simulink model "Engine"  (Simulink 9.2)
settings: Solver=ode23tb  StartTime=0.0  StopTime=50  FixedStep=0.001  EnableMultiTasking=on
values from neighbouring files (symbols this model uses):
  a0 = 1.1647e-05    [EngineData.m]
  a1 = 3.0718e-05    [EngineData.m]
  a2 = 0.0029    [EngineData.m]
  dP_thrREF = 10000    [EngineData.m]
  KpThr = 2.0000e-07    (= 2e-07)    [EngineData.m]
  KpWg = 2.0000e-07    (= 2e-07)    [EngineData.m]
  n_r = 2    [EngineData.m]
  r_c = 9.5000    (= 9.5)    [EngineData.m]
  T_z = [0 1 2 3 4 5 6 7 8 9 10 11 ... (401 elements, 401x1)]    [EUDC_MAN.mat]    (also in FTP75_MAN.mat = [0 1 2 3 4 5 6 7 8 9 10 11 ... (1875 elements, 1875x1)]; WLTP_MAN.mat = [0 1 2 3 4 5 6 7 8 9 10 11 ... (1801 elements, 1801x1)])
  TiThr = 1.0000e-04    (= 0.0001)    [EngineData.m]
  TiWg = 1.0000e-04    (= 0.0001)    [EngineData.m]
  toggle_paf = toggle(2)    [RunEngine.m]
  toggle_vol = toggle(3)    [RunEngine.m]
  toggle_Waf = toggle(4)    [RunEngine.m]
  toggle_Wc = toggle(5)    [RunEngine.m]
  toggle_Wic = toggle(6)    [RunEngine.m]
  toggle_Wth = toggle(7)    [RunEngine.m]
  toggle_xth = toggle(8)    [RunEngine.m]
  toggle_ypic = toggle(9)    [RunEngine.m]
  toggle_ypim = toggle(10)    [RunEngine.m]
  toggle_yTic = toggle(11)    [RunEngine.m]
  toggle_yWaf = toggle(12)    [RunEngine.m]
undefined symbols (not defined in the file or in its folder): Newton, Raphson, TC_ENGINE
libraries: simulink x3
(part 2 of 3)

== system Engine/Generic Single-Turbocharged Engine/Intake Manifold Control Volume ==
  note: Ideal Gas
      | Law
  note: Energy
      | Balance
  note: Mass
      | Balance
  note: p
  mFlow up : Inport
  T up : Inport  Port=2
  Q in : Inport  Port=3
  T down : Inport  Port=4
  mFlow down : Inport  Port=5
  Constant1 : Constant  Value=R
  Constant2 : Constant  Value=R
  Constant3 : Constant  Value=V
  H_in : Product  Inputs=3  SaturateOnIntegerOverflow=on  InputSameDT=on  OutDataTypeStr=Inherit: Same as first input
  H_out : Product  Inputs=3  SaturateOnIntegerOverflow=on  InputSameDT=on  OutDataTypeStr=Inherit: Same as first input
  H_out1 : Product  Inputs=*/  SaturateOnIntegerOverflow=on  InputSameDT=on  OutDataTypeStr=Inherit: Same as first input
  Receiver Mass : Integrator  InitialCondition=p_init*V/R/T_init  ZeroCross=off
  Receiver Temperature : Integrator  InitialCondition=T_init  ZeroCross=off
  Sum : Sum  Inputs=++|  SaturateOnIntegerOverflow=on  InputSameDT=on  OutDataTypeStr=Inherit: Same as first input
  Sum1 : Sum  Inputs=+-|  SaturateOnIntegerOverflow=on  InputSameDT=on  OutDataTypeStr=Inherit: Same as first input
  Sum2 : Sum  Inputs=+-+-  SaturateOnIntegerOverflow=on  InputSameDT=on  OutDataTypeStr=Inherit: Same as first input
  c_v : Constant  Value=R/(gamma-1)
  m*R*T/V : Product  Inputs=***/  SaturateOnIntegerOverflow=on  InputSameDT=on  OutDataTypeStr=Inherit: Same as first input
  m*c_v : Product  SaturateOnIntegerOverflow=on  InputSameDT=on  OutDataTypeStr=Inherit: Same as first input
  mFlow*c_v*T : Product  Inputs=3  SaturateOnIntegerOverflow=on  InputSameDT=on  OutDataTypeStr=Inherit: Same as first input
  T : Outport
  p : Outport  Port=2
  wires:
  mFlow*c_v*T/1 -> Sum2/4
  c_v/1 -> mFlow*c_v*T/1, m*c_v/1, Sum/2  "c_v"
  Sum1/1 -> mFlow*c_v*T/2, Receiver Mass/1
  Receiver Temperature/1 -> mFlow*c_v*T/3, m*R*T/V/1, T/1
  Constant2/1 -> m*R*T/V/2
  Constant3/1 -> m*R*T/V/4
  m*R*T/V/1 -> p/1
  H_out1/1 -> Receiver Temperature/1
  m*c_v/1 -> H_out1/2
  Sum2/1 -> H_out1/1
  Q in/1 -> Sum2/3
  H_out/1 -> Sum2/2
  H_in/1 -> Sum2/1
  mFlow up/1 -> Sum1/1, H_in/2
  mFlow down/1 -> H_out/2, Sum1/2
  T down/1 -> H_out/1
  T up/1 -> H_in/1
  Constant1/1 -> Sum/1
  Sum/1 -> H_out/3, H_in/3  "c_p"
  Receiver Mass/1 -> m*R*T/V/3, m*c_v/2

== system Engine/Generic Single-Turbocharged Engine/Intercooler Control Volume ==
  note: Ideal Gas
      | Law
  note: Energy
      | Balance
  note: Mass
      | Balance
  note: p
  mFlow up : Inport
  T up : Inport  Port=2
  Q in : Inport  Port=3
  T down : Inport  Port=4
  mFlow down : Inport  Port=5
  Constant1 : Constant  Value=R
  Constant2 : Constant  Value=R
  Constant3 : Constant  Value=V
  H_in : Product  Inputs=3  SaturateOnIntegerOverflow=on  InputSameDT=on  OutDataTypeStr=Inherit: Same as first input
  H_out : Product  Inputs=3  SaturateOnIntegerOverflow=on  InputSameDT=on  OutDataTypeStr=Inherit: Same as first input
  H_out1 : Product  Inputs=*/  SaturateOnIntegerOverflow=on  InputSameDT=on  OutDataTypeStr=Inherit: Same as first input
  Receiver Mass : Integrator  InitialCondition=p_init*V/R/T_init  ZeroCross=off
  Receiver Temperature : Integrator  InitialCondition=T_init  LowerSaturationLimit=0  ZeroCross=off
  Sum : Sum  Inputs=++|  SaturateOnIntegerOverflow=on  InputSameDT=on  OutDataTypeStr=Inherit: Same as first input
  Sum1 : Sum  Inputs=+-|  SaturateOnIntegerOverflow=on  InputSameDT=on  OutDataTypeStr=Inherit: Same as first input
  Sum2 : Sum  Inputs=+-+-  SaturateOnIntegerOverflow=on  InputSameDT=on  OutDataTypeStr=Inherit: Same as first input
  c_v : Constant  Value=R/(gamma-1)
  m*R*T/V : Product  Inputs=***/  SaturateOnIntegerOverflow=on  InputSameDT=on  OutDataTypeStr=Inherit: Same as first input
  m*c_v : Product  SaturateOnIntegerOverflow=on  InputSameDT=on  OutDataTypeStr=Inherit: Same as first input
  mFlow*c_v*T : Product  Inputs=3  SaturateOnIntegerOverflow=on  InputSameDT=on  OutDataTypeStr=Inherit: Same as first input
  T : Outport
  p : Outport  Port=2
  wires:
  mFlow*c_v*T/1 -> Sum2/4
  c_v/1 -> mFlow*c_v*T/1, m*c_v/1, Sum/2  "c_v"
  Sum1/1 -> mFlow*c_v*T/2, Receiver Mass/1
  Receiver Temperature/1 -> mFlow*c_v*T/3, m*R*T/V/1, T/1
  Constant2/1 -> m*R*T/V/2
  Constant3/1 -> m*R*T/V/4
  m*R*T/V/1 -> p/1
  H_out1/1 -> Receiver Temperature/1
  m*c_v/1 -> H_out1/2
  Sum2/1 -> H_out1/1
  Q in/1 -> Sum2/3
  H_out/1 -> Sum2/2
  H_in/1 -> Sum2/1
  mFlow up/1 -> Sum1/1, H_in/2
  mFlow down/1 -> H_out/2, Sum1/2
  T down/1 -> H_out/1
  T up/1 -> H_in/1
  Constant1/1 -> Sum/1
  Sum/1 -> H_out/3, H_in/3  "c_p"
  Receiver Mass/1 -> m*R*T/V/3, m*c_v/2

== system Engine/Generic Single-Turbocharged Engine/Intercooler Incompressible Restriction and Temperature model ==
  T_cool [K] : Inport
  p_up : Inport  Port=2
  T_up : Inport  Port=3
  T_down : Inport  Port=4
  p_down : Inport  Port=5
  Intercooler Temperature Simple : Subsystem  mask(Intercooler temperature){}
      mask help:
      | Intercooler temperature drop model using intercooler
      | efficiency, epsilon.
      |    T_out=T_in-epsilon*(T_in-T_cool)
      mask Help:
      | Enter the value for epsilon and the block will calculate
      | the temperature out for the
  Intercooler Flow : Subsystem  mask(Restriction Incompressible Flow){H=TC_ENGINE.interCooler.H, p_lin=TC_ENGINE.interCooler.p_lin}
      mask prompts: H "Flow resistance"; p_lin "Linearization limit [Pa]"
      mask help:
      | Flow restriction for incompressible flows.
      |
      | The flow is modelled using the following function for the pressure drop over the system where the conditions refer to upstream conditions.
      |
      | delta p=H mFlow^2 T_in/p_in
      mask Help:
      | <h3>Flow restriction for incompressible flows.</h3>
      | <br>
      | The flow is modelled using the following function for the pressure drop over the system where the conditions refer to upstream conditions.
      | <br>
      | delta p=H mFlow^2 T_in/p_in
  Saturation : Saturate  UpperLimit=1  LowerLimit=0  ZeroCross=off
  epsilon : Constant  Value=TC_ENGINE.interCooler.epsilon
  W_ic : Outport
  T_fwd_flow [K] : Outport  Port=2
  wires:
  Intercooler Flow/1(m flow) -> W_ic/1
  p_up/1 -> Intercooler Flow/1(p up)
  T_up/1 -> Intercooler Flow/2(T up)
  T_down/1 -> Intercooler Flow/3(T down)
  p_down/1 -> Intercooler Flow/4(p down)
  T_cool [K]/1 -> Intercooler Temperature Simple/2(T_cool)
  Intercooler Temperature Simple/1(T_out) -> T_fwd_flow [K]/1
  Intercooler Flow/2(T flow) -> Intercooler Temperature Simple/1(T_in)
  epsilon/1 -> Saturation/1  "epsilon"
  Saturation/1 -> Intercooler Temperature Simple/3(epsilon)

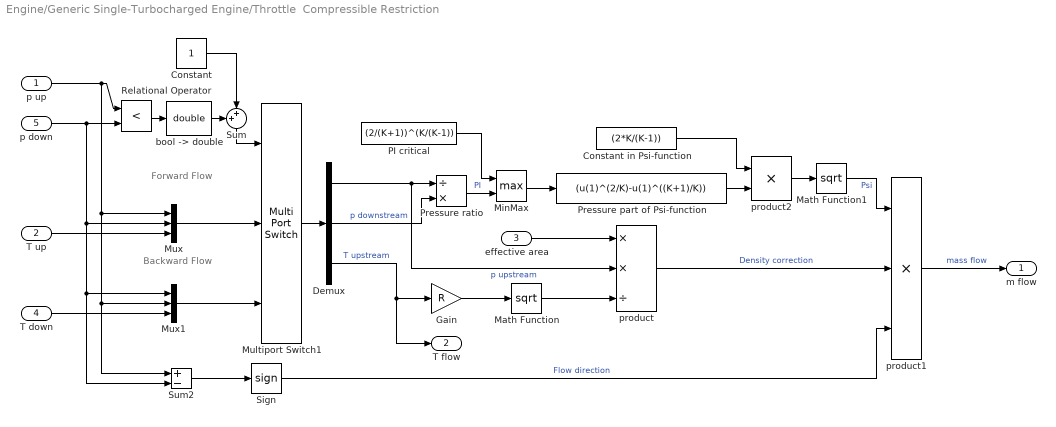
== system Engine/Generic Single-Turbocharged Engine/Throttle  Compressible Restriction ==
  note: Forward
      | Flow
  note: Backward
      | Flow
  p up : Inport
  T up : Inport  Port=2
  effective area : Inport  Port=3
  T down : Inport  Port=4
  p down : Inport  Port=5
  Constant : Constant
  Constant in Psi-function : Constant  Value=(2*K/(K-1))
  Demux : Demux  Outputs=3
  Gain : Gain  Gain=R  SaturateOnIntegerOverflow=on  OutDataTypeStr=Inherit: Same as input  ParamDataTypeStr=Inherit: Same as input
  Math Function : Math  Operator=sqrt  SaturateOnIntegerOverflow=on
  Math Function1 : Math  Operator=sqrt  SaturateOnIntegerOverflow=on
  MinMax : MinMax  Function=max  Inputs=2  ZeroCross=off  SaturateOnIntegerOverflow=on  InputSameDT=on
  Multiport Switch1 : MultiPortSwitch  Inputs=2  SaturateOnIntegerOverflow=on  InputSameDT=on
  Mux : Mux  Inputs=3
  Mux1 : Mux  Inputs=3
  PI critical : Constant  Value=(2/(K+1))^(K/(K-1))
  Pressure ratio : Product  Inputs=/*  SaturateOnIntegerOverflow=on  InputSameDT=on  OutDataTypeStr=Inherit: Same as first input
  Pressure part of Psi-function : Fcn  Expr=(u(1)^(2/K)-u(1)^((K+1)/K))
  Relational Operator : RelationalOperator  Operator=<  RndMeth=Nearest  InputSameDT=on
  Sign : Signum  ZeroCross=off
  Sum : Sum  Inputs=++|  SaturateOnIntegerOverflow=on  InputSameDT=on  OutDataTypeStr=Inherit: Same as first input
  Sum2 : Sum  Inputs=+-  SaturateOnIntegerOverflow=on  InputSameDT=on  OutDataTypeStr=Inherit: Same as first input
  "bool -> double" : DataTypeConversion  OutDataTypeStr=double  SaturateOnIntegerOverflow=on  RndMeth=Zero
  product : Product  Inputs=**/  SaturateOnIntegerOverflow=on  InputSameDT=on  OutDataTypeStr=Inherit: Same as first input
  product1 : Product  Inputs=3  SaturateOnIntegerOverflow=on  InputSameDT=on  OutDataTypeStr=Inherit: Same as first input
  product2 : Product  SaturateOnIntegerOverflow=on  InputSameDT=on  OutDataTypeStr=Inherit: Same as first input
  m flow : Outport
  T flow : Outport  Port=2
  wires:
  "bool -> double"/1 -> Sum/1
  Demux/3 -> T flow/1, Gain/1  "T upstream"
  Math Function1/1 -> product1/1  "Psi"
  product2/1 -> Math Function1/1
  Sign/1 -> product1/3  "Flow direction"
  product/1 -> product1/2  "Density correction"
  Pressure part of Psi-function/1 -> product2/2
  Constant in Psi-function/1 -> product2/1
  Math Function/1 -> product/3
  Gain/1 -> Math Function/1
  Demux/1 -> product/2, Pressure ratio/1  "p upstream"
  effective area/1 -> product/1
  product1/1 -> m flow/1  "mass flow"
  MinMax/1 -> Pressure part of Psi-function/1
  PI critical/1 -> MinMax/1
  Pressure ratio/1 -> MinMax/2  "PI"
  Sum2/1 -> Sign/1
  Demux/2 -> Pressure ratio/2  "p downstream"
  p up/1 -> Sum2/1, Mux1/2, Mux/1, Relational Operator/1
  p down/1 -> Sum2/2, Mux1/1, Mux/2, Relational Operator/2
  T up/1 -> Mux/3
  T down/1 -> Mux1/3
  Mux/1 -> Multiport Switch1/2
  Sum/1 -> Multiport Switch1/1
  Constant/1 -> Sum/2
  Mux1/1 -> Multiport Switch1/3
  Multiport Switch1/1 -> Demux/1
  Relational Operator/1 -> "bool -> double"/1

== system Engine/Generic Single-Turbocharged Engine/Turbine Control Volume ==
  note: Ideal Gas
      | Law
  note: Energy
      | Balance
  note: Mass
      | Balance
  note: p
  mFlow up : Inport
  T up : Inport  Port=2
  Q in : Inport  Port=3
  T down : Inport  Port=4
  mFlow down : Inport  Port=5
  Constant1 : Constant  Value=R
  Constant2 : Constant  Value=R
  Constant3 : Constant  Value=V
  H_in : Product  Inputs=3  SaturateOnIntegerOverflow=on  InputSameDT=on  OutDataTypeStr=Inherit: Same as first input
  H_out : Product  Inputs=3  SaturateOnIntegerOverflow=on  InputSameDT=on  OutDataTypeStr=Inherit: Same as first input
  H_out1 : Product  Inputs=*/  SaturateOnIntegerOverflow=on  InputSameDT=on  OutDataTypeStr=Inherit: Same as first input
  Receiver Mass : Integrator  InitialCondition=p_init*V/R/T_init  UpperSaturationLimit=500  LowerSaturationLimit=0  ZeroCross=off
  Receiver Temperature : Integrator  InitialCondition=T_init  UpperSaturationLimit=2000  LowerSaturationLimit=0  ZeroCross=off
  Sum : Sum  Inputs=++|  SaturateOnIntegerOverflow=on  InputSameDT=on  OutDataTypeStr=Inherit: Same as first input
  Sum1 : Sum  Inputs=+-|  SaturateOnIntegerOverflow=on  InputSameDT=on  OutDataTypeStr=Inherit: Same as first input
  Sum2 : Sum  Inputs=+-+-  SaturateOnIntegerOverflow=on  InputSameDT=on  OutDataTypeStr=Inherit: Same as first input
  c_v : Constant  Value=R/(gamma-1)
  m*R*T/V : Product  Inputs=***/  SaturateOnIntegerOverflow=on  InputSameDT=on  OutDataTypeStr=Inherit: Same as first input
  m*c_v : Product  SaturateOnIntegerOverflow=on  InputSameDT=on  OutDataTypeStr=Inherit: Same as first input
  mFlow*c_v*T : Product  Inputs=3  SaturateOnIntegerOverflow=on  InputSameDT=on  OutDataTypeStr=Inherit: Same as first input
  T : Outport
  p : Outport  Port=2
  wires:
  mFlow*c_v*T/1 -> Sum2/4
  c_v/1 -> mFlow*c_v*T/1, m*c_v/1, Sum/2  "c_v"
  Sum1/1 -> mFlow*c_v*T/2, Receiver Mass/1
  Receiver Temperature/1 -> mFlow*c_v*T/3, m*R*T/V/1, T/1
  Constant2/1 -> m*R*T/V/2
  Constant3/1 -> m*R*T/V/4
  m*R*T/V/1 -> p/1
  H_out1/1 -> Receiver Temperature/1
  m*c_v/1 -> H_out1/2
  Sum2/1 -> H_out1/1
  Q in/1 -> Sum2/3
  H_out/1 -> Sum2/2
  H_in/1 -> Sum2/1
  mFlow up/1 -> Sum1/1, H_in/2
  mFlow down/1 -> H_out/2, Sum1/2
  T down/1 -> H_out/1
  T up/1 -> H_in/1
  Constant1/1 -> Sum/1
  Sum/1 -> H_out/3, H_in/3  "c_p"
  Receiver Mass/1 -> m*R*T/V/3, m*c_v/2

== system Engine/Generic Single-Turbocharged Engine/Turbine and wastegate ==
  p_t : Inport
  T_t : Inport  Port=2
  w_tc : Inport  Port=3
  u_wg : Inport  Port=4
  p_em : Inport  Port=5
  T_em : Inport  Port=6
  A_wg : Gain  Gain=TC_ENGINE.wastegate.Amax*TC_ENGINE.wastegate.Cd  SaturateOnIntegerOverflow=on  OutDataTypeStr=Inherit: Same as input  ParamDataTypeStr=Inherit: Same as input
  A_wg2 : Gain  Gain=-1  SaturateOnIntegerOverflow=on  OutDataTypeStr=Inherit: Same as input  ParamDataTypeStr=Inherit: Same as input
  Adiabatic mixer : Subsystem  mask(Adiabatic mixer){c_p1=TC_ENGINE.gasProp.exh.cp, c_p2=TC_ENGINE.gasProp.exh.cp}
      mask prompts: c_p1 "Specific heats flow 1 [J/kg K]"; c_p2 "Specific heats flow 2 [J/kg K]"
  Turbine1 : Subsystem
  Wastegate : Subsystem  mask(Restriction - Compressible Flow){K=TC_ENGINE.gasProp.exh.kappa, R=TC_ENGINE.gasProp.exh.R}
      mask prompts: K "Ratio of specific heats"; R "Ideal gas constant [J/kg/ K]"
      mask help:
      | The flow is modelled using isentropic expansion in a nozzle with the assumption that there is no pressure recovery after the nozzle.
      |
      | See e.g. Heywood Appendix C for a derivation.
      mask Help:
      | <h3>Flow restriction for compressible flows.</h3>
      | <br>
      | The flow is modelled using isentropic expansion in a nozzle with the assumption that there is no pressure recovery after the nozzle.
      | 
      | See e.g. Heywood Appendix C for a derivation.
  T_turb : Outport
  W_es : Outport  Port=2
  Tq_t : Outport  Port=3
  wires:
  Wastegate/1(m flow) -> Adiabatic mixer/4(mFlow2)
  Wastegate/2(T flow) -> Adiabatic mixer/3(T2)
  A_wg/1 -> Wastegate/3(effective area)
  w_tc/1 -> Turbine1/1(w_tc [rad/s])
  p_t/1 -> Turbine1/2(p_t [Pa]), Wastegate/5(p down)
  p_em/1 -> Turbine1/3(p_em [Pa]), Wastegate/1(p up)
  T_em/1 -> Turbine1/4(T_em [K]), Wastegate/2(T up)
  u_wg/1 -> A_wg/1
  Adiabatic mixer/1(T mix) -> T_turb/1
  Adiabatic mixer/2(m tot) -> A_wg2/1
  Turbine1/3(W_t [kg/s]) -> Adiabatic mixer/2(mFlow1)
  Turbine1/1(Tq_t [Nm]) -> Tq_t/1
  Turbine1/2(T_t [K]) -> Adiabatic mixer/1(T1)
  T_t/1 -> Wastegate/4(T down)
  A_wg2/1 -> W_es/1

== system Engine/Generic Single-Turbocharged Engine/Waf Fault ==
  Tamb : Inport
  pamb : Inport  Port=2
  "pc " : Inport  Port=3
  Constant in Psi-function : Constant  Value=(2*K/(K-1))
  Manual Switch : ManualSwitch
  Math Function : Math  Operator=sqrt  SaturateOnIntegerOverflow=on
  Math Function1 : Math  SaturateOnIntegerOverflow=on
  MinMax : MinMax  Function=max  Inputs=2  ZeroCross=off  SaturateOnIntegerOverflow=on  InputSameDT=on
  PI critical : Constant  Value=(2/(K+1))^(K/(K-1))
  Pressure ratio : Product  Inputs=*/  SaturateOnIntegerOverflow=on  InputSameDT=on  OutDataTypeStr=Inherit: Same as first input
  Pressure part of Psi-function : Fcn  Expr=(u(1)^(2/K)-u(1)^((K+1)/K))
  Ramp : simulink/Sources/Ramp  slope=1/(2/3*T_z(end))  start=200  InitialOutput=0
  Saturation : Saturate  UpperLimit=inf  LowerLimit=0
  Step : Step  Time=0.3*size(T_z,1)  SampleTime=0
  To Workspace2 : ToWorkspace  VariableName=fWafSig  SaveFormat=Timeseries  SampleTime=-1
  product : Product  Inputs=*/*  SaturateOnIntegerOverflow=on  InputSameDT=on  OutDataTypeStr=Inherit: Same as first input
  product1 : Product  SaturateOnIntegerOverflow=on  InputSameDT=on  OutDataTypeStr=Inherit: Same as first input
  product2 : Product  SaturateOnIntegerOverflow=on  InputSameDT=on  OutDataTypeStr=Inherit: Same as first input
  "toggle " : Gain  Gain=toggle_Waf*10e-6  SaturateOnIntegerOverflow=on  OutDataTypeStr=Inherit: Same as input  ParamDataTypeStr=Inherit: Same as input
  fWaf : Outport
  wires:
  Tamb/1 -> Math Function/1  "T upstream"
  Math Function1/1 -> product1/1  "Psi"
  product2/1 -> Math Function1/1
  product/1 -> product1/2  "Density correction"
  Pressure part of Psi-function/1 -> product2/2
  Constant in Psi-function/1 -> product2/1
  pamb/1 -> Pressure ratio/1, product/1  "p upstream"
  MinMax/1 -> Pressure part of Psi-function/1
  PI critical/1 -> MinMax/1
  Pressure ratio/1 -> MinMax/2  "PI"
  Math Function/1 -> product/2
  "toggle "/1 -> product/3, To Workspace2/1
  "pc "/1 -> Pressure ratio/2
  product1/1 -> fWaf/1
  Ramp/1 -> Saturation/1
  Step/1 -> Manual Switch/2
  Saturation/1 -> Manual Switch/1
  Manual Switch/1 -> "toggle "/1

== system Engine/Generic Single-Turbocharged Engine/Wc Fault ==
  "pic " : Inport
  pamb : Inport  Port=2
  Tamb : Inport  Port=3
  Constant in Psi-function : Constant  Value=(2*K/(K-1))
  Math Function : Math  Operator=sqrt  SaturateOnIntegerOverflow=on
  Math Function1 : Math  Operator=sqrt  SaturateOnIntegerOverflow=on
  MinMax : MinMax  Function=max  Inputs=2  ZeroCross=off  SaturateOnIntegerOverflow=on  InputSameDT=on
  PI critical : Constant  Value=(2/(K+1))^(K/(K-1))
  Pressure ratio : Product  Inputs=*/  SaturateOnIntegerOverflow=on  InputSameDT=on  OutDataTypeStr=Inherit: Same as first input
  Pressure part of Psi-function : Fcn  Expr=(u(1)^(2/K)-u(1)^((K+1)/K))
  Step : Step  Time=0.4*size(T_z,1)  SampleTime=0
  To Workspace2 : ToWorkspace  VariableName=fWcSig  SaveFormat=Timeseries  SampleTime=-1
  product : Product  Inputs=*/*  SaturateOnIntegerOverflow=on  InputSameDT=on  OutDataTypeStr=Inherit: Same as first input
  product1 : Product  SaturateOnIntegerOverflow=on  InputSameDT=on  OutDataTypeStr=Inherit: Same as first input
  product2 : Product  SaturateOnIntegerOverflow=on  InputSameDT=on  OutDataTypeStr=Inherit: Same as first input
  "toggle " : Gain  Gain=toggle_Wc*3e-6  SaturateOnIntegerOverflow=on  OutDataTypeStr=Inherit: Same as input  ParamDataTypeStr=Inherit: Same as input
  fWc : Outport
  wires:
  Tamb/1 -> Math Function/1  "T upstream"
  Math Function1/1 -> product1/1  "Psi"
  product2/1 -> Math Function1/1
  product/1 -> product1/2  "Density correction"
  Pressure part of Psi-function/1 -> product2/2
  Constant in Psi-function/1 -> product2/1
  pamb/1 -> Pressure ratio/1, product/1  "p upstream"
  MinMax/1 -> Pressure part of Psi-function/1
  PI critical/1 -> MinMax/1
  Pressure ratio/1 -> MinMax/2  "PI"
  Math Function/1 -> product/2
  "toggle "/1 -> To Workspace2/1, product/3
  "pic "/1 -> Pressure ratio/2
  product1/1 -> fWc/1
  Step/1 -> "toggle "/1

== system Engine/Generic Single-Turbocharged Engine/Wic Fault ==
  "pic " : Inport
  pamb : Inport  Port=2
  Tamb : Inport  Port=3
  Constant in Psi-function : Constant  Value=(2*K/(K-1))
  Math Function : Math  Operator=sqrt  SaturateOnIntegerOverflow=on
  Math Function1 : Math  Operator=sqrt  SaturateOnIntegerOverflow=on
  MinMax : MinMax  Function=max  Inputs=2  ZeroCross=off  SaturateOnIntegerOverflow=on  InputSameDT=on
  PI critical : Constant  Value=(2/(K+1))^(K/(K-1))
  Pressure ratio : Product  Inputs=*/  SaturateOnIntegerOverflow=on  InputSameDT=on  OutDataTypeStr=Inherit: Same as first input
  Pressure part of Psi-function : Fcn  Expr=(u(1)^(2/K)-u(1)^((K+1)/K))
  Product1 : Product
  Step : Step  Time=0.4*size(T_z,1)  SampleTime=0
  Step1 : Step  Time=0.8*size(T_z,1)  Before=1  After=0  SampleTime=0
  To Workspace2 : ToWorkspace  VariableName=fWicSig  SaveFormat=Timeseries  SampleTime=-1
  product : Product  Inputs=*/*  SaturateOnIntegerOverflow=on  InputSameDT=on  OutDataTypeStr=Inherit: Same as first input
  product1 : Product  SaturateOnIntegerOverflow=on  InputSameDT=on  OutDataTypeStr=Inherit: Same as first input
  product2 : Product  SaturateOnIntegerOverflow=on  InputSameDT=on  OutDataTypeStr=Inherit: Same as first input
  "toggle " : Gain  Gain=toggle_Wic*10e-6  SaturateOnIntegerOverflow=on  OutDataTypeStr=Inherit: Same as input  ParamDataTypeStr=Inherit: Same as input
  fWic : Outport
  wires:
  Tamb/1 -> Math Function/1  "T upstream"
  Math Function1/1 -> product1/1  "Psi"
  product2/1 -> Math Function1/1
  product/1 -> product1/2  "Density correction"
  Pressure part of Psi-function/1 -> product2/2
  Constant in Psi-function/1 -> product2/1
  pamb/1 -> Pressure ratio/1, product/1  "p upstream"
  MinMax/1 -> Pressure part of Psi-function/1
  PI critical/1 -> MinMax/1
  Pressure ratio/1 -> MinMax/2  "PI"
  Math Function/1 -> product/2
  "toggle "/1 -> To Workspace2/1, product/3
  "pic "/1 -> Pressure ratio/2
  product1/1 -> fWic/1
  Product1/1 -> "toggle "/1
  Step/1 -> Product1/1
  Step1/1 -> Product1/2

== system Engine/Generic Single-Turbocharged Engine/Wth Fault ==
  pim : Inport
  Tamb : Inport  Port=2
  pamb : Inport  Port=3
  Constant in Psi-function : Constant  Value=(2*K/(K-1))
  Math Function : Math  Operator=sqrt  SaturateOnIntegerOverflow=on
  Math Function1 : Math  Operator=sqrt  SaturateOnIntegerOverflow=on
  MinMax : MinMax  Function=max  Inputs=2  ZeroCross=off  SaturateOnIntegerOverflow=on  InputSameDT=on
  PI critical : Constant  Value=(2/(K+1))^(K/(K-1))
  Pressure ratio : Product  Inputs=*/  SaturateOnIntegerOverflow=on  InputSameDT=on  OutDataTypeStr=Inherit: Same as first input
  Pressure part of Psi-function : Fcn  Expr=(u(1)^(2/K)-u(1)^((K+1)/K))
  Pulse Generator : DiscretePulseGenerator  PulseType=Time based  Period=200  PulseWidth=20  PhaseDelay=30
  To Workspace2 : ToWorkspace  VariableName=fWthSig  SaveFormat=Timeseries  SampleTime=-1
  product : Product  Inputs=*/*  SaturateOnIntegerOverflow=on  InputSameDT=on  OutDataTypeStr=Inherit: Same as first input
  product1 : Product  SaturateOnIntegerOverflow=on  InputSameDT=on  OutDataTypeStr=Inherit: Same as first input
  product2 : Product  SaturateOnIntegerOverflow=on  InputSameDT=on  OutDataTypeStr=Inherit: Same as first input
  "toggle " : Gain  Gain=toggle_Wth*1e-6  Multiplication=Matrix(K*u)  SaturateOnIntegerOverflow=on  OutDataTypeStr=Inherit: Same as input  ParamDataTypeStr=Inherit: Same as input
  fWth : Outport
  wires:
  Pulse Generator/1 -> "toggle "/1
  Tamb/1 -> Math Function/1  "T upstream"
  Math Function1/1 -> product1/1  "Psi"
  product2/1 -> Math Function1/1
  product/1 -> product1/2  "Density correction"
  Pressure part of Psi-function/1 -> product2/2
  Constant in Psi-function/1 -> product2/1
  pamb/1 -> Pressure ratio/2, product/1  "p upstream"
  MinMax/1 -> Pressure part of Psi-function/1
  PI critical/1 -> MinMax/1
  Pressure ratio/1 -> MinMax/2  "PI"
  Math Function/1 -> product/2
  "toggle "/1 -> To Workspace2/1, product/3
  pim/1 -> Pressure ratio/1
  product1/1 -> fWth/1

== system Engine/Generic Single-Turbocharged Engine/fyWaf Fault ==
  yWaf : Inport
  Product : Product
  Pulse Generator : DiscretePulseGenerator  PulseType=Time based  Period=150  PulseWidth=20  PhaseDelay=30
  Switch : Switch  Criteria=u2 > Threshold  ZeroCross=off
  To Workspace2 : ToWorkspace  VariableName=fyWafSig  SaveFormat=Timeseries  SampleTime=-1
  "toggle " : Gain  Gain=toggle_yWaf*1.2  SaturateOnIntegerOverflow=on  OutDataTypeStr=Inherit: Same as input  ParamDataTypeStr=Inherit: Same as input
  fyWaf : Outport
  wires:
  yWaf/1 -> Switch/3, Product/1
  "toggle "/1 -> Product/2, To Workspace2/1
  Pulse Generator/1 -> "toggle "/1
  Product/1 -> Switch/1, Switch/2
  Switch/1 -> fyWaf/1

== system Engine/Generic Single-Turbocharged Engine/yTic Fault ==
  yTic : Inport
  Pulse Generator : DiscretePulseGenerator  PulseType=Time based  Period=150  PulseWidth=20  PhaseDelay=30
  Sum : Sum  Inputs=|++
  To Workspace2 : ToWorkspace  VariableName=fyTicSig  SaveFormat=Timeseries  SampleTime=-1
  "toggle " : Gain  Gain=toggle_yTic*(-20)  SaturateOnIntegerOverflow=on  OutDataTypeStr=Inherit: Same as input  ParamDataTypeStr=Inherit: Same as input
  fyTic : Outport
  wires:
  yTic/1 -> Sum/1
  "toggle "/1 -> To Workspace2/1, Sum/2
  Pulse Generator/1 -> "toggle "/1
  Sum/1 -> fyTic/1

== system Engine/Generic Single-Turbocharged Engine/ypic Fault ==
  ypic : Inport
  Product : Product
  Pulse Generator : DiscretePulseGenerator  PulseType=Time based  Period=200  PulseWidth=20  PhaseDelay=30
  Switch : Switch  Criteria=u2 > Threshold  ZeroCross=off
  To Workspace2 : ToWorkspace  VariableName=fypicSig  SaveFormat=Timeseries  SampleTime=-1
  "toggle " : Gain  Gain=toggle_ypic*1.2  SaturateOnIntegerOverflow=on  OutDataTypeStr=Inherit: Same as input  ParamDataTypeStr=Inherit: Same as input
  fypic : Outport
  wires:
  ypic/1 -> Switch/3, Product/1
  "toggle "/1 -> Product/2, To Workspace2/1
  Product/1 -> Switch/1, Switch/2
  Switch/1 -> fypic/1
  Pulse Generator/1 -> "toggle "/1

== system Engine/Generic Single-Turbocharged Engine/ypim Fault ==
  ypim : Inport
  Manual Switch : ManualSwitch
  Product : Product
  Pulse Generator : DiscretePulseGenerator  PulseType=Time based  Period=120  PulseWidth=10  PhaseDelay=30
  Ramp : simulink/Sources/Ramp  slope=1/(2/3*T_z(end))  start=200  InitialOutput=0
  Saturation : Saturate  UpperLimit=inf  LowerLimit=0
  Switch : Switch  Criteria=u2 > Threshold  ZeroCross=off
  To Workspace2 : ToWorkspace  VariableName=fypimSig  SaveFormat=Timeseries  SampleTime=-1
  "toggle " : Gain  Gain=toggle_ypim*1.19  SaturateOnIntegerOverflow=on  OutDataTypeStr=Inherit: Same as input  ParamDataTypeStr=Inherit: Same as input
  fypim : Outport
  wires:
  ypim/1 -> Product/1, Switch/3
  "toggle "/1 -> Product/2, To Workspace2/1
  Product/1 -> Switch/1, Switch/2
  Switch/1 -> fypim/1
  Ramp/1 -> Saturation/1
  Pulse Generator/1 -> Manual Switch/2
  Saturation/1 -> Manual Switch/1
  Manual Switch/1 -> "toggle "/1

== system Engine/Boost Controller/Subsystem/% -> Area ==
  % : Inport
  Constant : Constant  Value=3
  Gain : Gain  Gain=997
  Sum : Sum  Inputs=|++
  A : Outport
  wires:
  Sum/1 -> A/1
  Constant/1 -> Sum/2
  Gain/1 -> Sum/1
  %/1 -> Gain/1

== system Engine/Boost Controller/Throttle Feed Forward /Aeff2alpha ==
  Aeff_REF : Inport
  AeffMinMax : Saturate  UpperLimit=a0+a1+a2  LowerLimit=a0
  Divide : Product  Inputs=*/
  Divide1 : Product  Inputs=/*/
  Sqrt : Sqrt  AlgorithmType=Newton-Raphson  SaturateOnIntegerOverflow=on
  Sub : Sum  Inputs=+-
  Sub1 : Sum
  Sub2 : Sum  Inputs=+-
  a0 : Constant  Value=a0
  a1 : Constant  Value=a1
  a2 : Constant  Value=a2
  square : Math  Operator=square  SaturateOnIntegerOverflow=on
  two : Constant  Value=2
  alpha_REF : Outport
  wires:
  Aeff_REF/1 -> AeffMinMax/1
  a0/1 -> Sub/2
  Sub/1 -> Divide/1
  a2/1 -> Divide/2, Divide1/1
  a1/1 -> Divide1/2
  two/1 -> Divide1/3
  Divide/1 -> Sub1/1
  Divide1/1 -> Sub2/2, square/1
  Sub1/1 -> Sqrt/1
  Sqrt/1 -> Sub2/1
  Sub2/1 -> alpha_REF/1
  square/1 -> Sub1/2
  AeffMinMax/1 -> Sub/1

== system Engine/Boost Controller/Throttle Feed Forward /Cylinder air flow REF ==
  p_im_REF : Inport
  T_im [K] : Inport  Port=2
  N [rad/s] : Inport  Port=3
  "p_em " : Inport  Port=4
  H_in2 : Product  Inputs=****/  SaturateOnIntegerOverflow=on  InputSameDT=on  OutDataTypeStr=Inherit: Same as first input
  Other constants : Constant  Value=V_D/4/pi/TC_ENGINE.gasProp.air.R
  Pressure ratio : Product  Inputs=/*  SaturateOnIntegerOverflow=on  InputSameDT=on  OutDataTypeStr=Inherit: Same as first input
  Sum : Sum  Inputs=+-|  SaturateOnIntegerOverflow=on  InputSameDT=on  OutDataTypeStr=Inherit: Same as first input
  Volumetric efficiency constants : Constant  Value=0.8/(r_c-1)
  compression ratio : Constant  Value=r_c
  expansion : Fcn  Expr=u(1)^(1/TC_ENGINE.gasProp.exh.kappa)
  product of constants : Product  SaturateOnIntegerOverflow=on  InputSameDT=on  OutDataTypeStr=Inherit: Same as first input
  m_dot_ac_REF : Outport
  wires:
  "p_em "/1 -> Pressure ratio/2
  expansion/1 -> Sum/2
  Pressure ratio/1 -> expansion/1  "PI"
  p_im_REF/1 -> H_in2/1, Pressure ratio/1
  Sum/1 -> H_in2/2
  product of constants/1 -> H_in2/3
  N [rad/s]/1 -> H_in2/4
  T_im [K]/1 -> H_in2/5
  Other constants/1 -> product of constants/2
  Volumetric efficiency constants/1 -> product of constants/1
  compression ratio/1 -> Sum/1
  H_in2/1 -> m_dot_ac_REF/1

== system Engine/Boost Controller/Throttle Feed Forward /Psi(PI) ==
  PI : Inport
  (g+1)/g : Constant  Value=(TC_ENGINE.throttle.gamma+1)/TC_ENGINE.throttle.gamma
  2/g : Constant  Value=2/TC_ENGINE.throttle.gamma
  2g/(g-1) : Constant  Value=(2*TC_ENGINE.throttle.gamma)/(TC_ENGINE.throttle.gamma-1)
  DivZeroProtect : MinMax  Function=max  Inputs=2
  Math Function : Math  Operator=pow  SaturateOnIntegerOverflow=on
  Math Function1 : Math  Operator=pow  SaturateOnIntegerOverflow=on
  MinMax : MinMax  Function=max  Inputs=2
  PI critical (2/(g+1))^(g/(g-1)) : Constant  Value=(2/(TC_ENGINE.throttle.gamma+1))^(TC_ENGINE.throttle.gamma/(TC_ENGINE.throttle.gamma-1))
  Product : Product  RndMeth=Zero
  Sqrt : Sqrt  AlgorithmType=Newton-Raphson  SaturateOnIntegerOverflow=on
  Subtract : Sum  Inputs=+-
  "[0,1]" : Saturate  UpperLimit=1  LowerLimit=0
  eps : Constant  Value=eps
  Psi : Outport
  wires:
  PI/1 -> "[0,1]"/1  "PI"
  PI critical (2/(g+1))^(g/(g-1))/1 -> MinMax/2
  MinMax/1 -> Math Function/1, Math Function1/1  "PIlim"
  2/g/1 -> Math Function/2
  (g+1)/g/1 -> Math Function1/2
  "[0,1]"/1 -> MinMax/1
  Math Function/1 -> Subtract/1
  Math Function1/1 -> Subtract/2
  Subtract/1 -> Product/1
  2g/(g-1)/1 -> Product/2
  Product/1 -> Sqrt/1
  Sqrt/1 -> DivZeroProtect/1  "Psi"
  eps/1 -> DivZeroProtect/2
  DivZeroProtect/1 -> Psi/1

== system Engine/Generic Single-Turbocharged Engine/Air filter Incompressible Restriction/paf Fault ==
  H : Inport
  H_in2 : Product  SaturateOnIntegerOverflow=on  InputSameDT=on  OutDataTypeStr=Inherit: Same as first input
  Manual Switch : ManualSwitch
  Ramp : simulink/Sources/Ramp  slope=1/(2/3*T_z(end))  start=200  InitialOutput=0
  Saturation : Saturate  UpperLimit=inf  LowerLimit=0
  Step : Step  Time=0.15*size(T_z,1)  SampleTime=0
  Switch : Switch  Criteria=u2 > Threshold  ZeroCross=off
  To Workspace2 : ToWorkspace  VariableName=fpafSig  SaveFormat=Timeseries  SampleTime=-1
  "toggle " : Gain  Gain=toggle_paf*80  SaturateOnIntegerOverflow=on  OutDataTypeStr=Inherit: Same as input  ParamDataTypeStr=Inherit: Same as input
  fpaf : Outport
  wires:
  H_in2/1 -> To Workspace2/1, Switch/2, Switch/1
  H/1 -> Switch/3, H_in2/1
  Switch/1 -> fpaf/1
  "toggle "/1 -> H_in2/2
  Ramp/1 -> Saturation/1
  Step/1 -> Manual Switch/2
  Saturation/1 -> Manual Switch/1
  Manual Switch/1 -> "toggle "/1

== system Engine/Generic Single-Turbocharged Engine/Compressor/Compressor Example ==
  note: Downstream temperature is included
      | to give the same interface as an
      | implementation of surge capable
      | compressor model.
  p_af [Pa] : Inport
  T_in [K] : Inport  Port=2
  w_tc [rad/s] : Inport  Port=3
  T_ds : Inport  Port=4
  p_c [Pa] : Inport  Port=5
  Compressor Efficiency : Subsystem
  Compressor Mass Flow : Subsystem
  Compressor Temperature : Subsystem  mask(Compressor Temperature){gamma_c=1.4}
      mask prompts: gamma_c "Compressor gamma [-]"
      mask help:
      | Compressor temperature increase.
      | It is determined directly from the definition compressor
      | efficiency.
      mask Help:
      | Enter the value for the ratio of specific heat
      | for the compressor.
  Compressor Torque : Subsystem  mask(Compressor Torque){c_p=1100}
      mask prompts: c_p "Compressor c_p [J/kg K]"
      mask help:
      | Calculates the compressor torque.
      | It is calculated using the control volume analysis of a
      | compressor, where it is assumed that c_p is constant for
      | the compression process.
      mask Help: Enter the value for the specific heat c_p in the dialog box.
  PI-calc : Subsystem
  Terminator : Terminator
  W_c : Outport
  T_c [K] : Outport  Port=2
  Tq_c [Nm] : Outport  Port=3
  wires:
  T_ds/1 -> Terminator/1
  Compressor Torque/1(Tq_c) -> Tq_c [Nm]/1
  Compressor Temperature/1(T_out) -> T_c [K]/1, Compressor Torque/4(T_out)
  PI-calc/1(PI) -> Compressor Temperature/3(Pi_c)  "PI_c"
  p_af [Pa]/1 -> Compressor Mass Flow/2(p_in [Pa]), PI-calc/1(p_af), Compressor Efficiency/3(p_in [Pa])
  p_c [Pa]/1 -> PI-calc/2(p_c), Compressor Mass Flow/4(p_c [Pa])
  T_in [K]/1 -> Compressor Efficiency/4(T_in [K]), Compressor Temperature/2(T_in), Compressor Torque/3(T_in), Compressor Mass Flow/3(T_in [K])
  w_tc [rad/s]/1 -> Compressor Mass Flow/1(w_c [rad/s]), Compressor Efficiency/1(w_c [rad/s]), Compressor Torque/1(omega_c)
  Compressor Mass Flow/1(W_c) -> W_c/1, Compressor Efficiency/2(W_c [kg/s]), Compressor Torque/2(mFlow_c)
  Compressor Efficiency/1(eta_c) -> Compressor Temperature/1(eta_c)

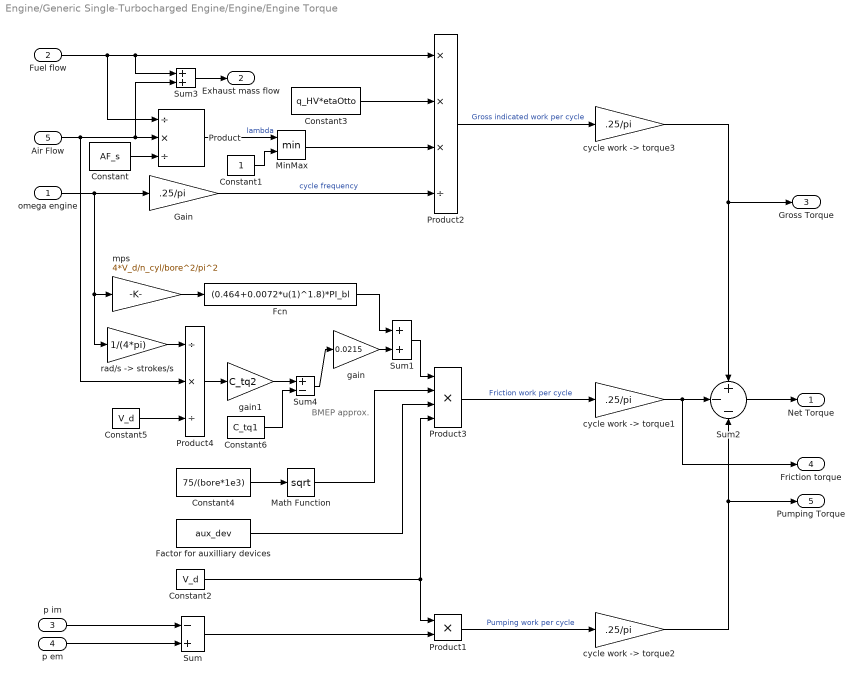
== system Engine/Generic Single-Turbocharged Engine/Engine/Engine Torque ==
  note: BMEP
      | approx.
  omega engine : Inport
  Fuel flow : Inport  Port=2
  p im : Inport  Port=3
  p em : Inport  Port=4
  Air Flow : Inport  Port=5
  Constant : Constant  Value=AF_s
  Constant1 : Constant
  Constant2 : Constant  Value=V_d
  Constant3 : Constant  Value=q_HV*etaOtto
  Constant4 : Constant  Value=75/(bore*1e3)
  Constant5 : Constant  Value=V_d
  Constant6 : Constant  Value=C_tq1
  Factor for auxilliary devices : Constant  Value=aux_dev
  Fcn : Fcn  Expr=(0.464+0.0072*u(1)^1.8)*PI_bl
  Gain : Gain  Gain=.25/pi  SaturateOnIntegerOverflow=on  OutDataTypeStr=Inherit: Same as input  ParamDataTypeStr=Inherit: Same as input
  Math Function : Math  Operator=sqrt  SaturateOnIntegerOverflow=on
  MinMax : MinMax  Inputs=2  ZeroCross=off  SaturateOnIntegerOverflow=on  InputSameDT=on
  Product : Product  Inputs=/*/  SaturateOnIntegerOverflow=on  InputSameDT=on  OutDataTypeStr=Inherit: Same as first input
  Product1 : Product  SaturateOnIntegerOverflow=on  InputSameDT=on  OutDataTypeStr=Inherit: Same as first input
  Product2 : Product  Inputs=***/  SaturateOnIntegerOverflow=on  InputSameDT=on  OutDataTypeStr=Inherit: Same as first input
  Product3 : Product  Inputs=4  SaturateOnIntegerOverflow=on  InputSameDT=on  OutDataTypeStr=Inherit: Same as first input
  Product4 : Product  Inputs=/*/  SaturateOnIntegerOverflow=on  InputSameDT=on  OutDataTypeStr=Inherit: Same as first input
  Sum : Sum  Inputs=-+  SaturateOnIntegerOverflow=on  InputSameDT=on  OutDataTypeStr=Inherit: Same as first input
  Sum1 : Sum  Inputs=2  SaturateOnIntegerOverflow=on  InputSameDT=on  OutDataTypeStr=Inherit: Same as first input
  Sum2 : Sum  Inputs=+--  SaturateOnIntegerOverflow=on  InputSameDT=on  OutDataTypeStr=Inherit: Same as first input
  Sum3 : Sum  Inputs=2  SaturateOnIntegerOverflow=on  InputSameDT=on  OutDataTypeStr=Inherit: Same as first input
  Sum4 : Sum  Inputs=+-  SaturateOnIntegerOverflow=on  InputSameDT=on  OutDataTypeStr=Inherit: Same as first input
  "cycle work -> torque1" : Gain  Gain=.25/pi  SaturateOnIntegerOverflow=on  OutDataTypeStr=Inherit: Same as input  ParamDataTypeStr=Inherit: Same as input
  "cycle work -> torque2" : Gain  Gain=.25/pi  SaturateOnIntegerOverflow=on  OutDataTypeStr=Inherit: Same as input  ParamDataTypeStr=Inherit: Same as input
  "cycle work -> torque3" : Gain  Gain=.25/pi  SaturateOnIntegerOverflow=on  OutDataTypeStr=Inherit: Same as input  ParamDataTypeStr=Inherit: Same as input
  gain : Gain  Gain=0.0215  SaturateOnIntegerOverflow=on  OutDataTypeStr=Inherit: Same as input  ParamDataTypeStr=Inherit: Same as input
  gain1 : Gain  Gain=C_tq2  SaturateOnIntegerOverflow=on  OutDataTypeStr=Inherit: Same as input  ParamDataTypeStr=Inherit: Same as input
  mps : Gain  Gain=4*V_d/n_cyl/bore^2/pi^2  SaturateOnIntegerOverflow=on  OutDataTypeStr=Inherit: Same as input  ParamDataTypeStr=Inherit: Same as input
  "rad/s -> strokes/s" : Gain  Gain=1/(4*pi)  SaturateOnIntegerOverflow=on  OutDataTypeStr=Inherit: Same as input  ParamDataTypeStr=Inherit: Same as input
  Net Torque : Outport
  Exhaust mass flow : Outport  Port=2
  Gross Torque : Outport  Port=3
  Friction torque : Outport  Port=4
  Pumping Torque : Outport  Port=5
  wires:
  gain1/1 -> Sum4/1
  Product4/1 -> gain1/1
  Sum4/1 -> gain/1
  Constant6/1 -> Sum4/2
  Constant5/1 -> Product4/3
  "rad/s -> strokes/s"/1 -> Product4/1
  Fcn/1 -> Sum1/1
  mps/1 -> Fcn/1
  Air Flow/1 -> Product4/2, Sum3/2, Product/2
  Fuel flow/1 -> Sum3/1, Product2/1, Product/1
  gain/1 -> Sum1/2
  Constant2/1 -> Product3/4, Product1/1
  Factor for auxilliary devices/1 -> Product3/3
  p im/1 -> Sum/1
  "cycle work -> torque2"/1 -> Pumping Torque/1, Sum2/3
  "cycle work -> torque1"/1 -> Friction torque/1, Sum2/2
  "cycle work -> torque3"/1 -> Gross Torque/1, Sum2/1
  Sum2/1 -> Net Torque/1
  Product2/1 -> "cycle work -> torque3"/1  "Gross indicated work per cycle"
  Product1/1 -> "cycle work -> torque2"/1  "Pumping work per cycle"
  Product3/1 -> "cycle work -> torque1"/1  "Friction work per cycle"
  Sum3/1 -> Exhaust mass flow/1
  Sum/1 -> Product1/2
  p em/1 -> Sum/2
  Constant4/1 -> Math Function/1
  Math Function/1 -> Product3/2
  Sum1/1 -> Product3/1
  omega engine/1 -> "rad/s -> strokes/s"/1, mps/1, Gain/1
  Constant1/1 -> MinMax/2
  Product/1 -> MinMax/1  "lambda"
  Constant/1 -> Product/3
  MinMax/1 -> Product2/3
  Constant3/1 -> Product2/2
  Gain/1 -> Product2/4  "cycle frequency"

== system Engine/Generic Single-Turbocharged Engine/Engine/Engine flow ==
  p im : Inport
  T im : Inport  Port=2
  omega engine : Inport  Port=3
  p em : Inport  Port=4
  Abs : Abs  ZeroCross=off
  H_in2 : Product  Inputs=****/  SaturateOnIntegerOverflow=on  InputSameDT=on  OutDataTypeStr=Inherit: Same as first input
  Other constants : Constant  Value=V_d/4/pi/R
  Pressure ratio : Product  Inputs=/*  SaturateOnIntegerOverflow=on  InputSameDT=on  OutDataTypeStr=Inherit: Same as first input
  Sum : Sum  Inputs=+-|  SaturateOnIntegerOverflow=on  InputSameDT=on  OutDataTypeStr=Inherit: Same as first input
  Volumetric Efficiency Fault : Subsystem
  Volumetric efficiency constants : Constant  Value=C/(r_c-1)
  compression ratio : Constant  Value=r_c
  expansion : Fcn  Expr=u(1)^(1/K)
  product of constants : Product  SaturateOnIntegerOverflow=on  InputSameDT=on  OutDataTypeStr=Inherit: Same as first input
  air mass flow : Outport
  wires:
  p em/1 -> Pressure ratio/2
  expansion/1 -> Sum/2
  Pressure ratio/1 -> Abs/1  "PI"
  p im/1 -> H_in2/1, Pressure ratio/1
  Sum/1 -> H_in2/2
  product of constants/1 -> H_in2/3
  omega engine/1 -> H_in2/4
  T im/1 -> H_in2/5
  H_in2/1 -> air mass flow/1
  Other constants/1 -> product of constants/2
  compression ratio/1 -> Sum/1
  Volumetric efficiency constants/1 -> Volumetric Efficiency Fault/1(Cvol)
  Volumetric Efficiency Fault/1(fCvol) -> product of constants/1
  Abs/1 -> expansion/1

== system Engine/Generic Single-Turbocharged Engine/Engine/Engine out temperature  (lambda=1) ==
  mass flow : Inport
  Constant : Constant  Value=T_0
  Gain : Gain  Gain=C  SaturateOnIntegerOverflow=on  OutDataTypeStr=Inherit: Same as input  ParamDataTypeStr=Inherit: Same as input
  Sum : Sum  Inputs=|++  SaturateOnIntegerOverflow=on  InputSameDT=on  OutDataTypeStr=Inherit: Same as first input
  T out : Outport
  wires:
  mass flow/1 -> Gain/1
  Sum/1 -> T out/1
  Constant/1 -> Sum/2
  Gain/1 -> Sum/1

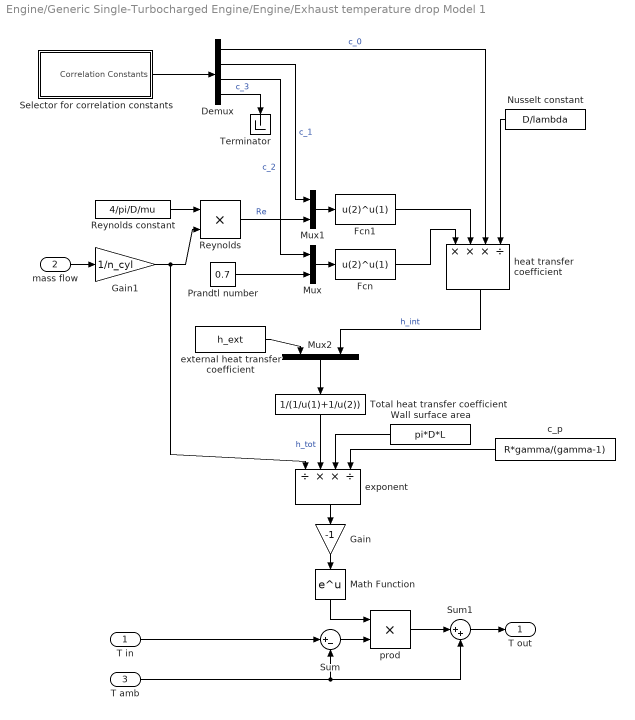
== system Engine/Generic Single-Turbocharged Engine/Engine/Exhaust temperature drop Model 1 ==
  T in : Inport
  mass flow : Inport  Port=2
  T amb : Inport  Port=3
  Demux : Demux
  Fcn : Fcn  Expr=u(2)^u(1)
  Fcn1 : Fcn  Expr=u(2)^u(1)
  Gain : Gain  Gain=-1  SaturateOnIntegerOverflow=on  OutDataTypeStr=Inherit: Same as input  ParamDataTypeStr=Inherit: Same as input
  Gain1 : Gain  Gain=1/n_cyl  SaturateOnIntegerOverflow=on  OutDataTypeStr=Inherit: Same as input  ParamDataTypeStr=Inherit: Same as input
  Math Function : Math  SaturateOnIntegerOverflow=on
  Mux : Mux  Inputs=2
  Mux1 : Mux  Inputs=2
  Mux2 : Mux  Inputs=2
  Nusselt constant : Constant  Value=D/lambda
  Prandtl number : Constant  Value=0.7
  Reynolds : Product  SaturateOnIntegerOverflow=on  InputSameDT=on  OutDataTypeStr=Inherit: Same as first input
  Reynolds constant : Constant  Value=4/pi/D/mu
  Selector for correlation constants : Subsystem
  Sum : Sum  Inputs=|+-  SaturateOnIntegerOverflow=on  InputSameDT=on  OutDataTypeStr=Inherit: Same as first input
  Sum1 : Sum  Inputs=|++  SaturateOnIntegerOverflow=on  InputSameDT=on  OutDataTypeStr=Inherit: Same as first input
  Terminator : Terminator
  Total heat transfer coefficient : Fcn  Expr=1/(1/u(1)+1/u(2))
  Wall surface area : Constant  Value=pi*D*L
  c_p : Constant  Value=R*gamma/(gamma-1)
  exponent : Product  Inputs=/**/  SaturateOnIntegerOverflow=on  InputSameDT=on  OutDataTypeStr=Inherit: Same as first input
  external heat transfer coefficient : Constant  Value=h_ext
  heat transfer coefficient : Product  Inputs=***/  SaturateOnIntegerOverflow=on  InputSameDT=on  OutDataTypeStr=Inherit: Same as first input
  prod : Product  SaturateOnIntegerOverflow=on  InputSameDT=on  OutDataTypeStr=Inherit: Same as first input
  T out : Outport
  wires:
  Selector for correlation constants/1(Correlation Constants) -> Demux/1
  Mux2/1 -> Total heat transfer coefficient/1
  Total heat transfer coefficient/1 -> exponent/2  "h_tot"
  exponent/1 -> Gain/1
  Math Function/1 -> prod/1
  Gain1/1 -> exponent/1, Reynolds/2
  mass flow/1 -> Gain1/1
  T amb/1 -> Sum1/2, Sum/2
  T in/1 -> Sum/1
  Sum1/1 -> T out/1
  prod/1 -> Sum1/1
  Sum/1 -> prod/2
  Fcn/1 -> heat transfer coefficient/1
  Prandtl number/1 -> Mux/2
  Mux/1 -> Fcn/1
  Gain/1 -> Math Function/1
  c_p/1 -> exponent/4
  heat transfer coefficient/1 -> Mux2/2  "h_int"
  external heat transfer coefficient/1 -> Mux2/1
  Wall surface area/1 -> exponent/3
  Demux/1 -> heat transfer coefficient/3  "c_0"
  Fcn1/1 -> heat transfer coefficient/2
  Nusselt constant/1 -> heat transfer coefficient/4
  Demux/3 -> Mux/1  "c_2"
  Mux1/1 -> Fcn1/1
  Reynolds constant/1 -> Reynolds/1
  Demux/2 -> Mux1/1  "c_1"
  Reynolds/1 -> Mux1/2  "Re"
  Demux/4 -> Terminator/1  "c_3"

== system Engine/Generic Single-Turbocharged Engine/Intercooler Incompressible Restriction and Temperature model/Intercooler Temperature Simple ==
  T_in : Inport
  T_cool : Inport  Port=2
  epsilon : Inport  Port=3
  Product : Product  SaturateOnIntegerOverflow=on  OutDataTypeStr=Inherit: Same as first input
  Sum2 : Sum  Inputs=+-  SaturateOnIntegerOverflow=on
  Sum3 : Sum  Inputs=+-  SaturateOnIntegerOverflow=on
  T_out : Outport
  wires:
  Sum3/1 -> T_out/1
  Sum2/1 -> Product/1
  T_in/1 -> Sum2/1, Sum3/1
  T_cool/1 -> Sum2/2
  Product/1 -> Sum3/2
  epsilon/1 -> Product/2

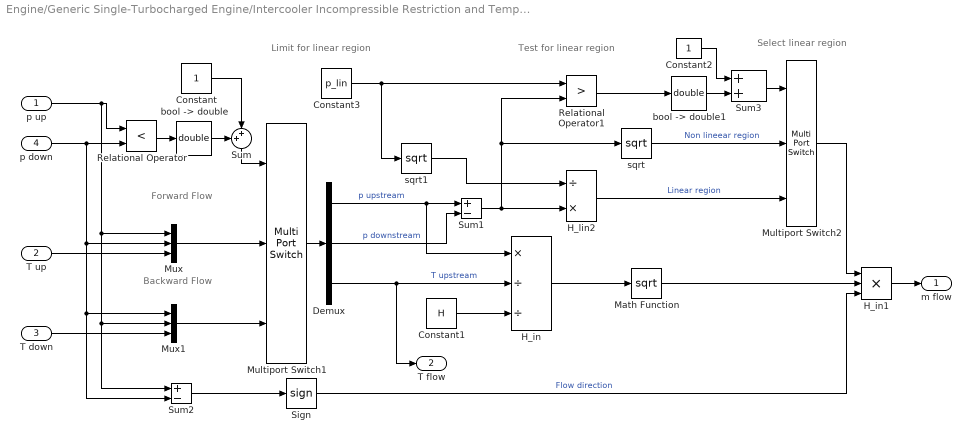
== system Engine/Generic Single-Turbocharged Engine/Intercooler Incompressible Restriction and Temperature model/Intercooler Flow ==
  note: Limit for linear region
  note: Select linear region
  note: Test for linear region
  note: Backward
      | Flow
  note: Forward
      | Flow
  p up : Inport
  T up : Inport  Port=2
  T down : Inport  Port=3
  p down : Inport  Port=4
  Constant : Constant
  Constant1 : Constant  Value=H
  Constant2 : Constant
  Constant3 : Constant  Value=p_lin
  Demux : Demux  Outputs=3
  H_in : Product  Inputs=*//  SaturateOnIntegerOverflow=on  InputSameDT=on  OutDataTypeStr=Inherit: Same as first input
  H_in1 : Product  Inputs=3  SaturateOnIntegerOverflow=on  InputSameDT=on  OutDataTypeStr=Inherit: Same as first input
  H_lin2 : Product  Inputs=/*  SaturateOnIntegerOverflow=on  InputSameDT=on  OutDataTypeStr=Inherit: Same as first input
  Math Function : Math  Operator=sqrt  SaturateOnIntegerOverflow=on
  Multiport Switch1 : MultiPortSwitch  Inputs=2  SaturateOnIntegerOverflow=on  InputSameDT=on
  Multiport Switch2 : MultiPortSwitch  Inputs=2  SaturateOnIntegerOverflow=on  InputSameDT=on
  Mux : Mux  Inputs=3
  Mux1 : Mux  Inputs=3
  Relational Operator : RelationalOperator  Operator=<  RndMeth=Nearest  InputSameDT=on
  Relational Operator1 : RelationalOperator  Operator=>  RndMeth=Nearest  InputSameDT=on
  Sign : Signum  ZeroCross=off
  Sum : Sum  Inputs=++|  SaturateOnIntegerOverflow=on  InputSameDT=on  OutDataTypeStr=Inherit: Same as first input
  Sum1 : Sum  Inputs=+-  SaturateOnIntegerOverflow=on  InputSameDT=on  OutDataTypeStr=Inherit: Same as first input
  Sum2 : Sum  Inputs=+-  SaturateOnIntegerOverflow=on  InputSameDT=on  OutDataTypeStr=Inherit: Same as first input
  Sum3 : Sum  Inputs=2  SaturateOnIntegerOverflow=on  InputSameDT=on  OutDataTypeStr=Inherit: Same as first input
  "bool -> double" : DataTypeConversion  OutDataTypeStr=double  SaturateOnIntegerOverflow=on  RndMeth=Zero
  "bool -> double1" : DataTypeConversion  OutDataTypeStr=double  SaturateOnIntegerOverflow=on  RndMeth=Zero
  sqrt : Math  Operator=sqrt  SaturateOnIntegerOverflow=on
  sqrt1 : Math  Operator=sqrt  SaturateOnIntegerOverflow=on
  m flow : Outport
  T flow : Outport  Port=2
  wires:
  "bool -> double1"/1 -> Sum3/2
  "bool -> double"/1 -> Sum/1
  Demux/3 -> T flow/1, H_in/2  "T upstream"
  Relational Operator1/1 -> "bool -> double1"/1
  Sign/1 -> H_in1/3  "Flow direction"
  Sum2/1 -> Sign/1
  Constant2/1 -> Sum3/1
  sqrt/1 -> Multiport Switch2/2  "Non lineear region"
  Constant3/1 -> Relational Operator1/1, sqrt1/1
  sqrt1/1 -> H_lin2/1
  Sum1/1 -> Relational Operator1/2, sqrt/1, H_lin2/2
  H_lin2/1 -> Multiport Switch2/3  "Linear region"
  H_in1/1 -> m flow/1
  Math Function/1 -> H_in1/2
  Multiport Switch2/1 -> H_in1/1
  Sum3/1 -> Multiport Switch2/1
  Relational Operator/1 -> "bool -> double"/1
  H_in/1 -> Math Function/1
  Constant1/1 -> H_in/3
  Demux/1 -> H_in/1, Sum1/1  "p upstream"
  Demux/2 -> Sum1/2  "p downstream"
  Multiport Switch1/1 -> Demux/1
  Mux1/1 -> Multiport Switch1/3
  Constant/1 -> Sum/2
  Sum/1 -> Multiport Switch1/1
  Mux/1 -> Multiport Switch1/2
  T down/1 -> Mux1/3
  T up/1 -> Mux/3
  p down/1 -> Relational Operator/2, Sum2/2, Mux1/1, Mux/2
  p up/1 -> Relational Operator/1, Sum2/1, Mux1/2, Mux/1

== system Engine/Generic Single-Turbocharged Engine/Turbine and wastegate/Adiabatic mixer ==
  T1 : Inport
  mFlow1 : Inport  Port=2
  T2 : Inport  Port=3
  mFlow2 : Inport  Port=4
  Constant : Constant  Value=c_p1
  Constant1 : Constant  Value=c_p2
  Product : Product  Inputs=3  SaturateOnIntegerOverflow=on  InputSameDT=on  OutDataTypeStr=Inherit: Same as first input
  Product1 : Product  Inputs=3  SaturateOnIntegerOverflow=on  InputSameDT=on  OutDataTypeStr=Inherit: Same as first input
  Product2 : Product  Inputs=*/  SaturateOnIntegerOverflow=on  InputSameDT=on  OutDataTypeStr=Inherit: Same as first input
  Product3 : Product  SaturateOnIntegerOverflow=on  InputSameDT=on  OutDataTypeStr=Inherit: Same as first input
  Product4 : Product  SaturateOnIntegerOverflow=on  InputSameDT=on  OutDataTypeStr=Inherit: Same as first input
  Sum : Sum  Inputs=2  SaturateOnIntegerOverflow=on  InputSameDT=on  OutDataTypeStr=Inherit: Same as first input
  Sum1 : Sum  Inputs=2  SaturateOnIntegerOverflow=on  InputSameDT=on  OutDataTypeStr=Inherit: Same as first input
  Sum2 : Sum  Inputs=2  SaturateOnIntegerOverflow=on  InputSameDT=on  OutDataTypeStr=Inherit: Same as first input
  T mix : Outport
  m tot : Outport  Port=2
  wires:
  Constant1/1 -> Product1/3, Product4/1
  mFlow2/1 -> Product4/2, Product1/2, Sum/2
  mFlow1/1 -> Product3/2, Product/2, Sum/1
  Constant/1 -> Product/3, Product3/1
  Product4/1 -> Sum2/2
  Product3/1 -> Sum2/1
  Product2/1 -> T mix/1
  Sum2/1 -> Product2/2
  Sum/1 -> m tot/1
  Sum1/1 -> Product2/1
  T2/1 -> Product1/1
  T1/1 -> Product/1
  Product1/1 -> Sum1/2
  Product/1 -> Sum1/1
